simulink model "rectifierfinal"  (R2015a)
settings: Solver=ode23tb  StartTime=0.0  StopTime=.1  RelTol=1e-3
libraries: powerlib x10
settings Model: Creator=binma  LastModifiedBy=binma

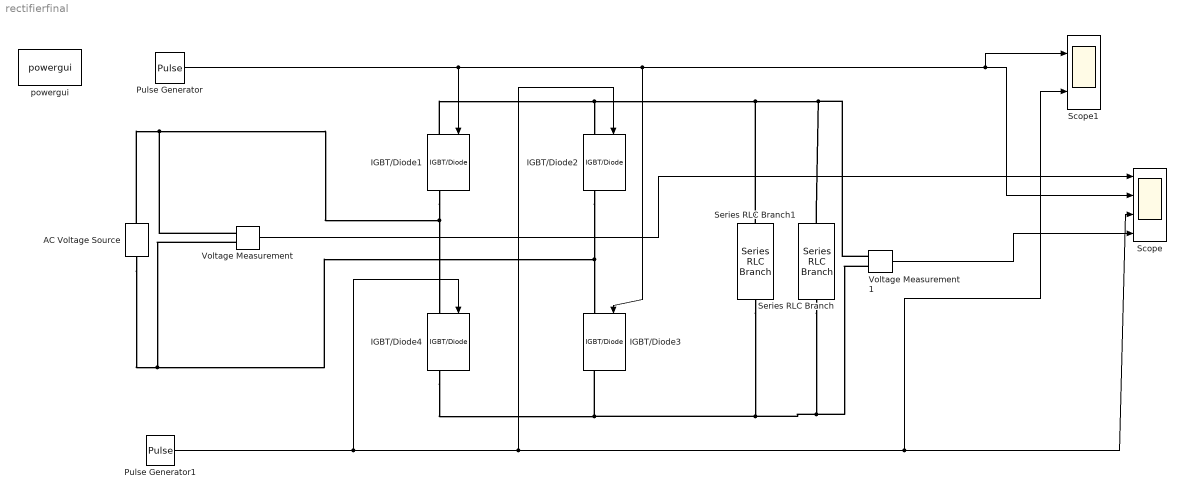
== system rectifierfinal ==
  AC Voltage Source : powerlib/Electrical Sources/AC Voltage Source  Amplitude=230  Phase=0  Frequency=50  SampleTime=0  Measurements=None
  IGBT/Diode{1..4} (4 alike) : powerlib/Power Electronics/IGBT//Diode  Ron=1e-3  Rs=1e5  Cs=inf  Measurements=on
  Pulse Generator : DiscretePulseGenerator  PulseType=Time based  Period=.02  PulseWidth=50
  Pulse Generator1 : DiscretePulseGenerator  PulseType=Time based  Period=.02  PulseWidth=50  PhaseDelay=0.01
  Scope : Scope  NumInputPorts=4
      settings: YMin=-1~-0~-1~-1  YMax=1~2~1~1
  Scope1 : Scope  NumInputPorts=2
      settings: YMin=-5~-5  YMax=5~5
  Series RLC Branch : powerlib/Elements/Series RLC Branch  LConnTagsString=__new0  RConnTagsString=__new0  BranchType=R  Resistance=1000  Inductance=1e-3  SetiL0=off  InitialCurrent=0  Capacitance=1e-6  Setx0=off  InitialVoltage=0  Measurements=None
  Series RLC Branch1 : powerlib/Elements/Series RLC Branch  LConnTagsString=__new0  RConnTagsString=__new0  BranchType=C  Resistance=1  Inductance=1e-3  SetiL0=off  InitialCurrent=0  Capacitance=800e-2  Setx0=off  InitialVoltage=0  Measurements=None
  Voltage Measurement : powerlib/Measurements/Voltage Measurement  PhasorSimulation=off  OutputType=Complex  PSBequivalent=0
  Voltage Measurement1 : powerlib/Measurements/Voltage Measurement  PhasorSimulation=off  OutputType=Complex  PSBequivalent=0
  powergui : powerlib/powergui  Priority=1  SimulationMode=Continuous  SolverType=Tustin/Backward Euler (TBE)  SampleTime=50e-6  frequency=60  SPID=off  DisableSnubberDevices=off  DisableRonSwitches=off  DisableVfSwitches=off  SwTol=0  DisplayEquations=off  Interpol=off  methode=off  Ts=100  FunctionMessages=off  echomessages=off  HookPort=off  EnableUseOfTLC=off  x0status=blocks  frequencyindice=50  Pbase=100e6  ErrMax=1e-4  Iterations=50  UnitsV=kV  UnitsW=MW  buscounter=0  RestoreLinks=warning  ResistiveCurrentMeasurement=off  Frange=[0:2:500]  Ylog=off  Xlog=on  ShowGrid=off  save=off  variable=ZData  structure=0  ZoomFFT=off  StartTime=0.0  cycles=1  DisplayStyle=1  fundamental=60  FreqAxis=off  MaxFrequency=1000  frequencyindicesteady=1  RmsSteady=1  display=off
  wires:
  Pulse Generator/1 -> IGBT/Diode1/1, IGBT/Diode3/1, Scope1/1, Scope/2
  Voltage Measurement/1 -> Scope/1
  Voltage Measurement1/1 -> Scope/4
  Pulse Generator1/1 -> IGBT/Diode4/1, IGBT/Diode2/1, Scope1/2, Scope/3
  connections:
  IGBT/Diode1/RConn1 -- Voltage Measurement/LConn1 -- AC Voltage Source/RConn1 -- IGBT/Diode4/LConn1
  IGBT/Diode2/RConn1 -- IGBT/Diode3/LConn1 -- AC Voltage Source/LConn1 -- Voltage Measurement/LConn2
  Series RLC Branch1/RConn1 -- IGBT/Diode4/RConn1 -- IGBT/Diode3/RConn1 -- Series RLC Branch/RConn1 -- Voltage Measurement1/LConn2
  IGBT/Diode1/LConn1 -- Voltage Measurement1/LConn1 -- Series RLC Branch/LConn1 -- Series RLC Branch1/LConn1 -- IGBT/Diode2/LConn1
